simulink model "equalizer_example_SIMULINK"  (R2023b)
settings: Solver=VariableStepAuto  StartTime=0.0  StopTime=180  RelTol=1e-3
libraries: simulink x3, audiosources x1, dspsnks4 x1, dspvision x1, audiofilters x1, dspsrcs4 x1, dspsigops x1
settings Model: Creator=macbookair  LastModifiedBy=macbookair

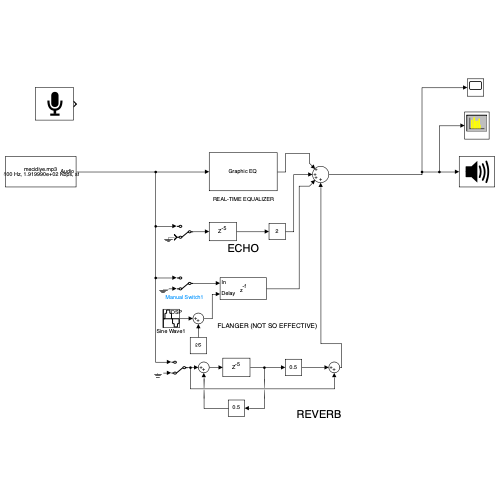
[thumbnail: Simulink's stored preview of the top-level diagram]
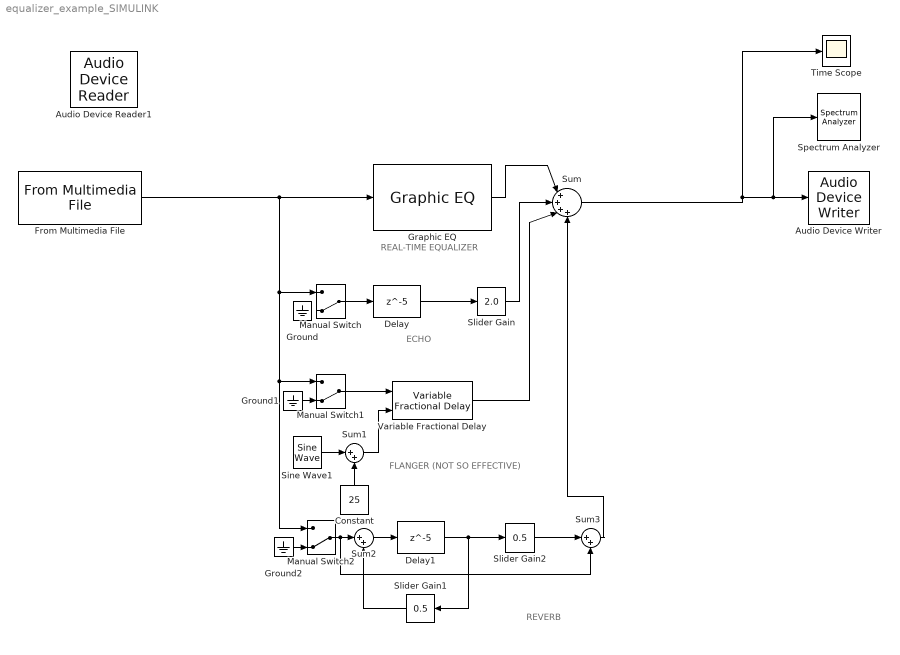
== system equalizer_example_SIMULINK ==
  note: REAL-TIME EQUALIZER
  note: ECHO
  note: FLANGER (NOT SO EFFECTIVE)
  note: REVERB
  Audio Device Reader1 : audiosources/Audio Device Reader  Driver=CoreAudio  Device=MacBook Air Microphone  SampleRate=44100  NumChannels=1  SamplesPerFrame=1024  BitDepth=16-bit integer  NumBuffers=10  DefaultInputChannelMapping=on  InputChannelMapping=1:2  OutputNumOverrunSamples=off  OutputDataType=double  DriverIdx=5  DeviceWarnFlag=''
  Audio Device Writer : dspsnks4/Audio Device Writer  Driver=CoreAudio  Device=OĞUZHAN's Buds2  InheritSampleRate=on  SampleRate=44100  BitDepth=16-bit integer  BufferSize=4096  NumBuffers=10  DefaultOutputChannelMapping=on  OutputChannelMapping=1:2  OutputNumUnderrunSamples=off  DriverIdx=5  DeviceWarnFlag=''
  Constant : Constant  Value=25
  Delay : Delay  DelayLength=5  DelayLengthUpperLimit=4000  InitialCondition=0
  Delay1 : Delay  DelayLength=5  DelayLengthUpperLimit=4000  InitialCondition=0
  From Multimedia File : dspvision/From Multimedia File  inputFilename=/Users/macbookair/Desktop/Projects/Matlab Things/EQUALIZER MUSIC PLAYER PROJECT/mecidiye.mp3  readRange=[1 Inf]  loop=on  numPlays=inf  outputStreams=Audio only  videoDataType=single  audioDataType=double  inheritSampleTime=on  userDefinedSampleTime=1/30  noAudioOutput=off  isIntensityVideo=off  fourcc=RGB  colorVideoFormat=Separate color signals  outputEOF=off  dataOrg=Column-major  audioFrameSize=1024  computeAudioFrameSize=off  outSamplingMode=Sample based
      settings: LibrarySourceBlock=audiosources/From Multimedia File
  Graphic EQ : audiofilters/Graphic EQ  EQOrder=2  Bandwidth=1 octave  Structure=Parallel  Gain_25=0  Gain_31_5=-20.0  Gain_40=0  Gain_50=0  Gain_63=-20.0  Gain_80=0  Gain_100=0  Gain_125=-18.400  Gain_160=0  Gain_200=0  Gain_250=-20.0  Gain_315=0  Gain_400=0  Gain_500=-20.0  Gain_630=0  Gain_800=0  Gain_1000=20.0  Gain_1250=0  Gain_1600=0  Gain_2000=20.0  Gain_2500=0  Gain_3150=0  Gain_4000=20.0  Gain_5000=0  Gain_6300=0  Gain_8000=-19.600  Gain_10000=0  Gain_12500=0  Gain_16000=20.0  Gain_20000=0  WorkspaceVariableName=myFilt  OverwriteExportVariable=on  InheritSampleRate=off  SampleRate=44100  SimulateUsing=Code generation
  Ground : Ground
  Ground1 : Ground
  Ground2 : Ground
  Manual Switch : ManualSwitch  CurrentSetting=0
  Manual Switch1 : ManualSwitch  CurrentSetting=0
  Manual Switch2 : ManualSwitch  CurrentSetting=0
  Sine Wave1 : dspsrcs4/Sine Wave  Amplitude=15  Frequency=0.5  Phase=0  SampleMode=Discrete  OutComplex=Real  CompMethod=Trigonometric fcn  TableSize=Speed  SampleTime=1/44100  SamplesPerFrame=1024  ResetState=Restart at time zero  OutputFrames=off  dataType=double  wordLen=16  udDataType=sfix(16)  fracBitsMode=Best precision  numFracBits=15  OutDataTypeStr=double  LastOutDataTypeStr=double
  Slider Gain : simulink/Math Operations/Slider Gain  gain=2.0  low=0  high=10
  Slider Gain1 : simulink/Math Operations/Slider Gain  gain=0.5  low=0  high=10
  Slider Gain2 : simulink/Math Operations/Slider Gain  gain=0.5  low=0  high=10
  Spectrum Analyzer : SpectrumAnalyzer  WindowPosition=[44.000000,72.000000,609.000000,472.000000,]  ScopeFrameLocation=window  SampleRateSource=Property  SampleRate=44.1e3  PlotAsTwoSidedSpectrum=off  FrequencyScale=Log  FrequencySpan=Start and stop frequencies  StartFrequency=20  StopFrequency=20e3  YLimits=[-98.84570227,28.44534587]
  Sum : Sum  Inputs=|++++
  Sum1 : Sum  Inputs=|++
  Sum2 : Sum  Inputs=|++
  Sum3 : Sum  Inputs=|++
  Time Scope : Scope
  Variable Fractional Delay : dspsigops/Variable Fractional Delay  mode=OBSOLETE  modeActive=Linear  L=4  FarrowL=4  R=10  alpha=1  dmax=5  InputProcessing=Columns as channels (frame based)  ic=0  noDFT=off  fallbackFIR=Clip to the minimum value necessary for centered kernel  fallbackFarrow=Clip to the minimum value necessary for centered kernel  roundingMode=Zero  overflowMode=off
  wires:
  Sum/1 -> Time Scope/1, Spectrum Analyzer/1, Audio Device Writer/1
  Delay/1 -> Slider Gain/1
  Slider Gain/1 -> Sum/2
  Graphic EQ/1 -> Sum/1
  Manual Switch/1 -> Delay/1
  From Multimedia File/1 -> Manual Switch1/1, Manual Switch2/1, Manual Switch/1, Graphic EQ/1
  Ground1/1 -> Manual Switch1/2
  Constant/1 -> Sum1/2
  Sum1/1 -> Variable Fractional Delay/2
  Variable Fractional Delay/1 -> Sum/3
  Sine Wave1/1 -> Sum1/1
  Manual Switch1/1 -> Variable Fractional Delay/1
  Manual Switch2/1 -> Sum3/2, Sum2/1
  Ground2/1 -> Manual Switch2/2
  Sum2/1 -> Delay1/1
  Slider Gain1/1 -> Sum2/2
  Delay1/1 -> Slider Gain2/1, Slider Gain1/1
  Slider Gain2/1 -> Sum3/1
  Sum3/1 -> Sum/4
